simulink model "tb_kinematics"  (R2024b)
settings: Solver=VariableStepAuto  StartTime=0.0  StopTime=8  RelTol=1e-3
undefined symbols (not defined in the file): eta, ki_tuner, kp_tuner, openloop, Ts_s
libraries: slpidlib x2, simulink x1
settings Model: PacingRate=1.100000  Creator=icpmoles  LastModifiedBy=icpmoles

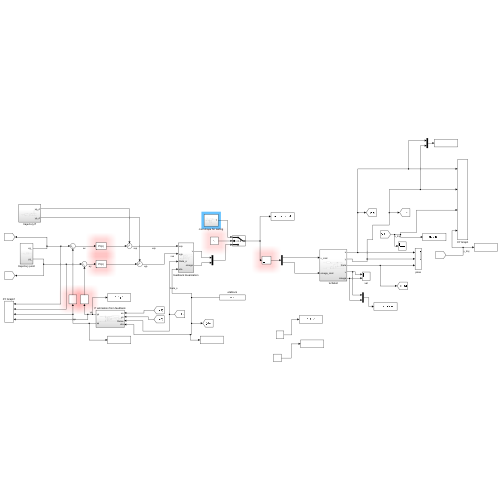
[thumbnail: Simulink's stored preview of the top-level diagram]
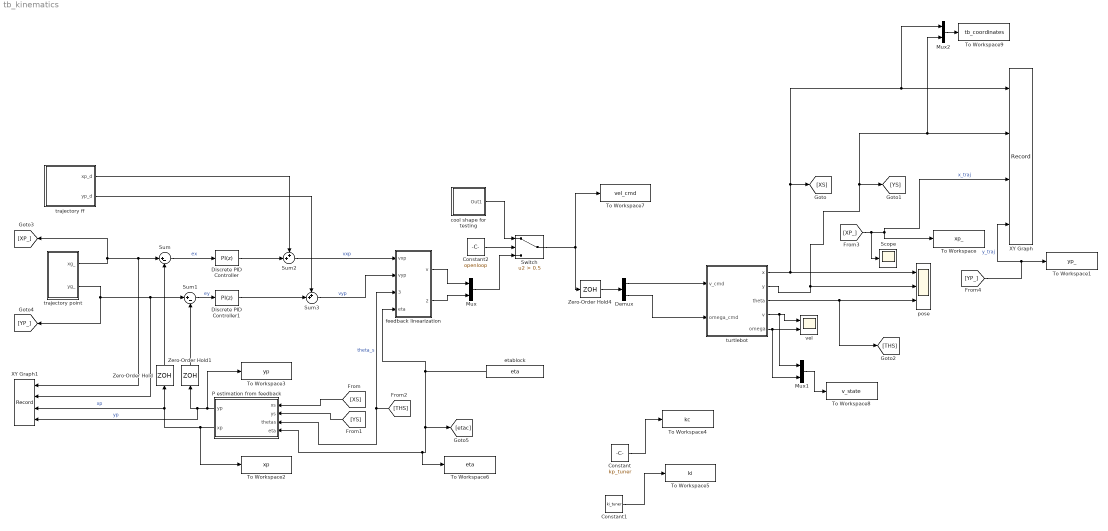
== system tb_kinematics ==
  Constant : Constant  Value=kp_tuner
  Constant1 : Constant  Value=ki_tuner
  Constant2 : Constant  Value=openloop
  Demux : Demux  Outputs=2
  Discrete PID Controller : slpidlib/PID Controller  Controller=PI  Form=Ideal  TimeDomain=Discrete-time  UseExternalTs=off  SampleTime=Ts_s  IntegratorMethod=Forward Euler  FilterMethod=Forward Euler  ControllerParametersSource=internal  P=kp_tuner  I=ki_tuner  UseKiTs=off  D=0  UseExternalDerivativeSource=off  N=100  UseFilter=on  TunerSelectOption=Transfer Function Based (PID Tuner App)  InitialConditionSource=internal  InitialConditionForIntegrator=0  InitialConditionForFilter=0  DifferentiatorICPrevScaledInput=0  ExternalReset=none  TrackingMode=off  Kt=1  LimitOutput=off  SatLimitsSource=internal  UpperSaturationLimit=inf  LowerSaturationLimit=-inf  LinearizeAsGain=off  AntiWindupMode=none  Kb=1  LimitIntegrator=off  UpperIntegratorSaturationLimit=inf  LowerIntegratorSaturationLimit=-inf  POutMin=[]  POutMax=[]  IOutMin=[]  IOutMax=[]  DOutMin=[]  DOutMax=[]  NOutMin=[]  NOutMax=[]  SumOutMin=[]  SumOutMax=[]  SaturationOutMin=[]  SaturationOutMax=[]  PParamMin=[]  PParamMax=[]  IParamMin=[]  IParamMax=[]  DParamMin=[]  DParamMax=[]  NParamMin=[]  NParamMax=[]  KbParamMin=[]  KbParamMax=[]  KtParamMin=[]  KtParamMax=[]  KbOutMin=[]  KbOutMax=[]  KtOutMin=[]  KtOutMax=[]  IntegratorOutMin=[]  IntegratorOutMax=[]  FilterOutMin=[]  FilterOutMax=[]  SumI1OutMin=[]  SumI1OutMax=[]  SumI2OutMin=[]  SumI2OutMax=[]  SumI3OutMin=[]  SumI3OutMax=[]  SumI4OutMin=[]  SumI4OutMax=[]  SumDOutMin=[]  SumDOutMax=[]  DifferentiatorOutMin=[]  DifferentiatorOutMax=[]  FilterDiffOutCoefMin=[]  FilterDiffOutCoefMax=[]  ReciprocalOutMin=[]  ReciprocalOutMax=[]  SumDenOutMin=[]  SumDenOutMax=[]  SumNumOutMin=[]  SumNumOutMax=[]  DivideOutMin=[]  DivideOutMax=[]  UdiffTsProdOutMin=[]  UdiffTsProdOutMax=[]  NTsProdOutMin=[]  NTsProdOutMax=[]  UintegralTsProdOutMin=[]  UintegralTsProdOutMax=[]  UngainTsProdOutMin=[]  UngainTsProdOutMax=[]  ClampingZeroOutDataTypeStr=Inherit: Inherit via back propagation  ClampingZeroOutMin=[]  ClampingZeroOutMax=[]  FilterDenConstantOutDataTypeStr=Inherit: Inherit via back propagation  FilterDenConstantOutMin=[]  FilterDenConstantOutMax=[]  PCopyOutDataTypeStr=Inherit: Inherit via back propagation  PCopyOutMin=[]  PCopyOutMax=[]  NCopyOutDataTypeStr=Inherit: Inherit via back propagation  NCopyOutMin=[]  NCopyOutMax=[]  IntegratorContinuousStateAttributes=''  IntegratorStateMustResolveToSignalObject=off  IntegratorRTWStateStorageClass=Auto  FilterContinuousStateAttributes=''  FilterStateMustResolveToSignalObject=off  FilterRTWStateStorageClass=Auto  ParallelPVariant=Passthrough  IdealPVariant=InternalParameters  IVariant=InternalParameters  DVariant=Disabled  IntegratorVariant=Discrete  SatVariant=Disabled  AWVariant=Passthrough  PCopyVariant=Disabled  TRVariant=Disabled  FdbkBlocksVariant=Forward  IdealPFdbkVariant=Disabled  SatFdbkVariant=Disabled  DerivativeFilterVariant=Disabled  NVariant=Disabled  NCopyVariant=Disabled_SignalSpec  FilterICVariant=Disabled  IntegratorICVariant=InternalICs  ExternalResetVariant=Disabled  TRSumVariant=Passthrough  SumFdbkVariant=Disabled  SumVariant=Sum_PI  TsampFilterVariant=InternalTs  TsampNgainVariant=Passthrough  TsampIntegralVariant=Disabled_SignalSpec  ExternalSaturationOutDataTypeStr=Inherit: Same as second input  DerivativeSourceVariant=Disabled  PreIntVariant=InternalPreInt
      settings: LibrarySourceBlock=hdlsllib/Discrete/Discrete PID Controller
  Discrete PID Controller1 : slpidlib/PID Controller  Controller=PI  Form=Ideal  TimeDomain=Discrete-time  UseExternalTs=off  SampleTime=Ts_s  IntegratorMethod=Forward Euler  FilterMethod=Forward Euler  ControllerParametersSource=internal  P=kp_tuner  I=ki_tuner  UseKiTs=off  D=0  UseExternalDerivativeSource=off  N=100  UseFilter=on  TunerSelectOption=Transfer Function Based (PID Tuner App)  InitialConditionSource=internal  InitialConditionForIntegrator=0  InitialConditionForFilter=0  DifferentiatorICPrevScaledInput=0  ExternalReset=none  TrackingMode=off  Kt=1  LimitOutput=off  SatLimitsSource=internal  UpperSaturationLimit=inf  LowerSaturationLimit=-inf  LinearizeAsGain=off  AntiWindupMode=none  Kb=1  LimitIntegrator=off  UpperIntegratorSaturationLimit=inf  LowerIntegratorSaturationLimit=-inf  POutMin=[]  POutMax=[]  IOutMin=[]  IOutMax=[]  DOutMin=[]  DOutMax=[]  NOutMin=[]  NOutMax=[]  SumOutMin=[]  SumOutMax=[]  SaturationOutMin=[]  SaturationOutMax=[]  PParamMin=[]  PParamMax=[]  IParamMin=[]  IParamMax=[]  DParamMin=[]  DParamMax=[]  NParamMin=[]  NParamMax=[]  KbParamMin=[]  KbParamMax=[]  KtParamMin=[]  KtParamMax=[]  KbOutMin=[]  KbOutMax=[]  KtOutMin=[]  KtOutMax=[]  IntegratorOutMin=[]  IntegratorOutMax=[]  FilterOutMin=[]  FilterOutMax=[]  SumI1OutMin=[]  SumI1OutMax=[]  SumI2OutMin=[]  SumI2OutMax=[]  SumI3OutMin=[]  SumI3OutMax=[]  SumI4OutMin=[]  SumI4OutMax=[]  SumDOutMin=[]  SumDOutMax=[]  DifferentiatorOutMin=[]  DifferentiatorOutMax=[]  FilterDiffOutCoefMin=[]  FilterDiffOutCoefMax=[]  ReciprocalOutMin=[]  ReciprocalOutMax=[]  SumDenOutMin=[]  SumDenOutMax=[]  SumNumOutMin=[]  SumNumOutMax=[]  DivideOutMin=[]  DivideOutMax=[]  UdiffTsProdOutMin=[]  UdiffTsProdOutMax=[]  NTsProdOutMin=[]  NTsProdOutMax=[]  UintegralTsProdOutMin=[]  UintegralTsProdOutMax=[]  UngainTsProdOutMin=[]  UngainTsProdOutMax=[]  ClampingZeroOutDataTypeStr=Inherit: Inherit via back propagation  ClampingZeroOutMin=[]  ClampingZeroOutMax=[]  FilterDenConstantOutDataTypeStr=Inherit: Inherit via back propagation  FilterDenConstantOutMin=[]  FilterDenConstantOutMax=[]  PCopyOutDataTypeStr=Inherit: Inherit via back propagation  PCopyOutMin=[]  PCopyOutMax=[]  NCopyOutDataTypeStr=Inherit: Inherit via back propagation  NCopyOutMin=[]  NCopyOutMax=[]  IntegratorContinuousStateAttributes=''  IntegratorStateMustResolveToSignalObject=off  IntegratorRTWStateStorageClass=Auto  FilterContinuousStateAttributes=''  FilterStateMustResolveToSignalObject=off  FilterRTWStateStorageClass=Auto  ParallelPVariant=Passthrough  IdealPVariant=InternalParameters  IVariant=InternalParameters  DVariant=Disabled  IntegratorVariant=Discrete  SatVariant=Disabled  AWVariant=Passthrough  PCopyVariant=Disabled  TRVariant=Disabled  FdbkBlocksVariant=Forward  IdealPFdbkVariant=Disabled  SatFdbkVariant=Disabled  DerivativeFilterVariant=Disabled  NVariant=Disabled  NCopyVariant=Disabled_SignalSpec  FilterICVariant=Disabled  IntegratorICVariant=InternalICs  ExternalResetVariant=Disabled  TRSumVariant=Passthrough  SumFdbkVariant=Disabled  SumVariant=Sum_PI  TsampFilterVariant=InternalTs  TsampNgainVariant=Passthrough  TsampIntegralVariant=Disabled_SignalSpec  ExternalSaturationOutDataTypeStr=Inherit: Same as second input  DerivativeSourceVariant=Disabled  PreIntVariant=InternalPreInt
      settings: LibrarySourceBlock=hdlsllib/Discrete/Discrete PID Controller
  Mux : Mux  Inputs=2
  Mux1 : Mux  Inputs=2
  Mux2 : Mux  Inputs=2
  P estimation from feedback : Subsystem
  Scope : Scope
  Sum : Sum  Inputs=|+-
  Sum1 : Sum  Inputs=|+-
  Sum2 : Sum  Inputs=++|
  Sum3 : Sum  Inputs=++|
  Switch : Switch  Criteria=u2 > Threshold  Threshold=0.5  SaturateOnIntegerOverflow=off  InputSameDT=off
  To Workspace : ToWorkspace  VariableName=xp_  SaveFormat=Timeseries  SampleTime=-1
  To Workspace1 : ToWorkspace  VariableName=yp_  SaveFormat=Timeseries  SampleTime=-1
  To Workspace2 : ToWorkspace  VariableName=xp  SaveFormat=Timeseries  SampleTime=-1
  To Workspace3 : ToWorkspace  VariableName=yp  SaveFormat=Timeseries  SampleTime=-1
  To Workspace4 : ToWorkspace  VariableName=kc  SaveFormat=Timeseries  SampleTime=-1
  To Workspace5 : ToWorkspace  VariableName=ki  SaveFormat=Timeseries  SampleTime=-1
  To Workspace6 : ToWorkspace  VariableName=eta  SaveFormat=Timeseries  SampleTime=-1
  To Workspace7 : ToWorkspace  VariableName=vel_cmd  SaveFormat=Timeseries  SampleTime=-1
  To Workspace8 : ToWorkspace  VariableName=v_state  SaveFormat=Timeseries  SampleTime=-1
  To Workspace9 : ToWorkspace  VariableName=tb_coordinates  SaveFormat=Timeseries  SampleTime=-1
  XY Graph : Record  FileSettingsInternal="{\"entries\":[{\"content\":{\"excelSettings\":{\"content\":{},\"type\":\"Streamout.ExcelSettings\"}},\"type\":\"Streamout.FileSettingStorage\",\"uuid\":\"\"}],\"packageUris\":[\"http:\\/\\/schema.mathworks.com\\/mf0\\/streamout_blocks\\/R2020a\"],\"version\":\"1.0\"}"  Layout=[1 1]  SignalsInternal="{\"entries\":[{\"content\":{\"signals\":[{\"content\":{\"blockPath\":[],\"dimensions\":[1],\"domain\":\"\",\"lineColor\":\"#a2142f\",\"plots\":[ 1 ],\"port\":1,\"sid\":[\"\"],\"signalID\":1,\"signalName\":\"turtlebot:1\"},\"type\":\"RecordBlkView.Signal\",\"uuid\":\"\"},{\"content\":{\"blockPath\":[],\"dimensions\":[1],\"domain\":\"\",\"lineColor\":\"#139fff\",\"plots\":[ 1 ],\"port\":2,\"sid\":[\"\"],\"signalID\":2,\"signalName\":\"turtlebot:2\"},\"type\":\"RecordBlkView.Signal\",\"uuid\":\"\"},{\"content\":{\"blockPath\":[],\"dimensions\":[1],\"domain\":\"\",\"lineColor\":\"#64d413\",\"lineWidth\":2,\"plots\":[ 1 ],\"port\":3,\"sid\":[\"\"],\"signalID\":3,\"signalName\":\"x_traj\"},\"type\":\"RecordBlkView.Signal\",\"uuid\":\"\"},{\"content\":{\"blockPath\":[],\"dimensions\":[1],\"domain\":\"\",\"lineColor\":\"#ff13a6\",\"lineWidth\":2,\"plots\":[ 1 ],\"port\":4,\"sid\":[\"\"],\"signalID\":4,\"signalName\":\"y_traj\"},\"type\":\"RecordBlkView.Signal\",\"uuid\":\"\"}]},\"type\":\"RecordBlkView.InputSignals\",\"uuid\":\"\"}],\"packageUris\":[\"http:\\/\\/schema.mathworks.com\\/mf0\\/streamout_blocks\\/R2020a\"],\"version\":\"1.0\"}"  VisualizationBindings="{\"xyplotplugin\":{\"info\":[{\"series\":[{\"bindingParametersList\":[{\"parameter\":\"X-Axis\",\"signalID\":1,\"signalName\":\"turtlebot:1\"},{\"parameter\":\"Y-Axis\",\"signalID\":2,\"signalName\":\"turtlebot:2\"}],\"seriesID\":0},{\"bindingParametersList\":[{\"parameter\":\"X-Axis\",\"signalID\":3,\"signalName\":\"x_traj\"},{\"parameter\":\"Y-Axis\",\"signalID\":4,\"signalName\":\"y_traj\"}],\"seriesID\":1}],\"subplotID\":1},{\"series\":[],\"subplotID\":9}]}}"  CompatibilityTag=XY
  XY Graph1 : Record  FileSettingsInternal="{\"entries\":[{\"content\":{\"excelSettings\":{\"content\":{},\"type\":\"Streamout.ExcelSettings\"}},\"type\":\"Streamout.FileSettingStorage\",\"uuid\":\"\"}],\"packageUris\":[\"http:\\/\\/schema.mathworks.com\\/mf0\\/streamout_blocks\\/R2020a\"],\"version\":\"1.0\"}"  Layout=[1 1]  SignalsInternal="{\"entries\":[{\"content\":{\"signals\":[{\"content\":{\"blockPath\":[],\"dimensions\":[1],\"domain\":\"\",\"lineColor\":\"#a2142f\",\"plots\":[ 1 ],\"port\":1,\"sid\":[\"\"],\"signalID\":1,\"signalName\":\"trajectory point:1\"},\"type\":\"RecordBlkView.Signal\",\"uuid\":\"\"},{\"content\":{\"blockPath\":[],\"dimensions\":[1],\"domain\":\"\",\"lineColor\":\"#139fff\",\"plots\":[ 1 ],\"port\":2,\"sid\":[\"\"],\"signalID\":2,\"signalName\":\"trajectory point:2\"},\"type\":\"RecordBlkView.Signal\",\"uuid\":\"\"},{\"content\":{\"blockPath\":[],\"dimensions\":[1],\"domain\":\"\",\"lineColor\":\"#edb120\",\"lineWidth\":2,\"plots\":[ 1 ],\"port\":3,\"sid\":[\"\"],\"signalID\":3,\"signalName\":\"xp\"},\"type\":\"RecordBlkView.Signal\",\"uuid\":\"\"},{\"content\":{\"blockPath\":[],\"dimensions\":[1],\"domain\":\"\",\"lineColor\":\"#7e2f8e\",\"lineWidth\":2,\"plots\":[ 1 ],\"port\":4,\"sid\":[\"\"],\"signalID\":4,\"signalName\":\"yp\"},\"type\":\"RecordBlkView.Signal\",\"uuid\":\"\"}]},\"type\":\"RecordBlkView.InputSignals\",\"uuid\":\"\"}],\"packageUris\":[\"http:\\/\\/schema.mathworks.com\\/mf0\\/streamout_blocks\\/R2020a\"],\"version\":\"1.0\"}"  VisualizationBindings="{\"xyplotplugin\":{\"info\":[{\"series\":[{\"bindingParametersList\":[{\"parameter\":\"X-Axis\",\"signalID\":1,\"signalName\":\"trajectory point:1\"},{\"parameter\":\"Y-Axis\",\"signalID\":2,\"signalName\":\"trajectory point:2\"}],\"seriesID\":0},{\"bindingParametersList\":[{\"parameter\":\"X-Axis\",\"signalID\":3,\"signalName\":\"xp\"},{\"parameter\":\"Y-Axis\",\"signalID\":4,\"signalName\":\"yp\"}],\"seriesID\":1}],\"subplotID\":1}]}}"  CompatibilityTag=XY
  Zero-Order Hold : ZeroOrderHold  SampleTime=Ts_s
  Zero-Order Hold1 : ZeroOrderHold  SampleTime=Ts_s
  Zero-Order Hold4 : ZeroOrderHold  SampleTime=Ts_s
  cool shape for testing : Subsystem
  etablock : Constant  Value=eta
  feedback linearization : Subsystem
  pose : Scope  NumInputPorts=3
  trajectory ff : Subsystem
  trajectory point : Subsystem
  turtlebot : Subsystem
  vel : Scope  NumInputPorts=2
  wires:
  turtlebot/1(x) -> [XS], Mux2/1, XY Graph/1, pose/1
  turtlebot/3(theta) -> [THS], pose/3
  turtlebot/4(v) -> Mux1/1, vel/1
  turtlebot/5(omega) -> Mux1/2, vel/2
  Demux/1 -> turtlebot/1(v_cmd)
  Demux/2 -> turtlebot/2(omega_cmd)
  P estimation from feedback/2(xp) -> To Workspace2/1, Zero-Order Hold/1, XY Graph1/3  "xp"
  P estimation from feedback/1(yp) -> To Workspace3/1, XY Graph1/4, Zero-Order Hold1/1  "yp"
  trajectory point/2(yg_) -> [YP_], XY Graph1/2, Sum1/1
  Sum/1 -> Discrete PID Controller/1  "ex"
  Sum1/1 -> Discrete PID Controller1/1  "ey"
  Discrete PID Controller1/1 -> Sum3/2
  Discrete PID Controller/1 -> Sum2/2
  [XS] -> P estimation from feedback/1(xs)
  [YS] -> P estimation from feedback/2(ys)
  [THS] -> P estimation from feedback/3(thetas), feedback linearization/3(theta_s)  "theta_s"
  Sum2/1 -> feedback linearization/1(vxp)  "vxp"
  Sum3/1 -> feedback linearization/2(vyp)  "vyp"
  etablock/1 -> [etac], To Workspace6/1, P estimation from feedback/4(eta), feedback linearization/4(eta)
  trajectory ff/2(yp_d) -> Sum3/1
  trajectory ff/1(xp_d) -> Sum2/1
  Zero-Order Hold/1 -> Sum/2
  Zero-Order Hold1/1 -> Sum1/2
  trajectory point/1(xg_) -> [XP_], XY Graph1/1, Sum/1
  [XP_] -> Scope/1, To Workspace/1, XY Graph/3  "x_traj"
  [YP_] -> XY Graph/4, To Workspace1/1  "y_traj"
  Constant/1 -> To Workspace4/1
  Constant1/1 -> To Workspace5/1
  feedback linearization/1(v) -> Mux/1
  feedback linearization/2(omega) -> Mux/2
  Constant2/1 -> Switch/2
  Zero-Order Hold4/1 -> Demux/1
  Mux/1 -> Switch/3
  cool shape for testing/1(Out1) -> Switch/1
  Mux1/1 -> To Workspace8/1
  Mux2/1 -> To Workspace9/1
  turtlebot/2(y) -> [YS], Mux2/2, XY Graph/2, pose/2
  Switch/1 -> Zero-Order Hold4/1, To Workspace7/1

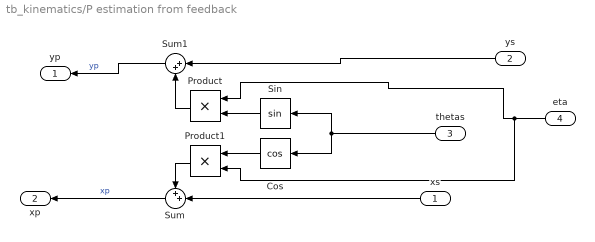
== system tb_kinematics/P estimation from feedback ==
  xs : Inport
  ys : Inport  Port=2
  thetas : Inport  Port=3
  eta : Inport  Port=4
  Cos : Trigonometry  Operator=cos
  Product : Product
  Product1 : Product
  Sin : Trigonometry
  Sum : Sum  Inputs=++|
  Sum1 : Sum  Inputs=|++
  yp : Outport
  xp : Outport  Port=2
  wires:
  xs/1 -> Sum/2
  thetas/1 -> Sin/1, Cos/1
  Sum/1 -> xp/1  "xp"
  Product1/1 -> Sum/1
  ys/1 -> Sum1/1
  Sin/1 -> Product/2
  Sum1/1 -> yp/1  "yp"
  Product/1 -> Sum1/2
  Cos/1 -> Product1/1
  eta/1 -> Product1/2, Product/1

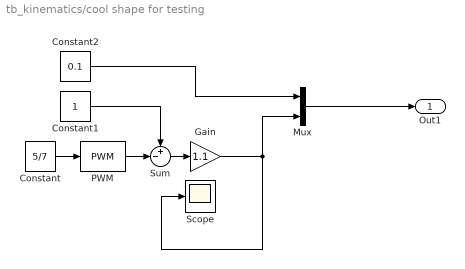
== system tb_kinematics/cool shape for testing ==
  Constant : Constant  Value=5/7
  Constant1 : Constant
  Constant2 : Constant  Value=0.1
  Gain : Gain  Gain=1.1
  Mux : Mux  Inputs=2
  PWM : simulink/Discontinuities/PWM  DisableCoverage=on  Period=7  InitialDelay=0  DisallowZeroDutyCycle=off  RunAtFixedTimeIntervals=off  SampleTime=0.1
  Scope : Scope
  Sum : Sum  Inputs=+-|
  Out1 : Outport
  wires:
  PWM/1 -> Sum/2
  Gain/1 -> Mux/2, Scope/1
  Constant1/1 -> Sum/1
  Constant/1 -> PWM/1
  Constant2/1 -> Mux/1
  Sum/1 -> Gain/1
  Mux/1 -> Out1/1

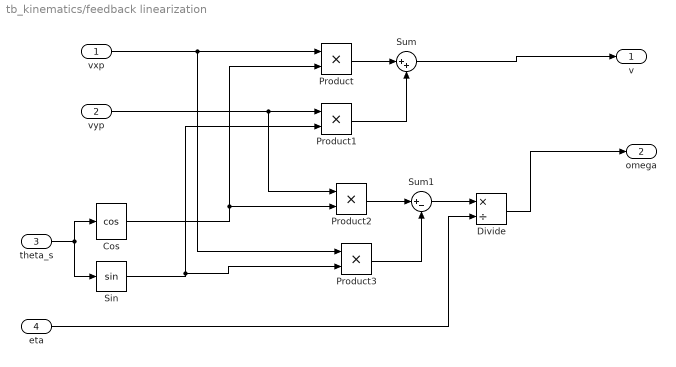
== system tb_kinematics/feedback linearization ==
  vxp : Inport
  vyp : Inport  Port=2
  theta_s : Inport  Port=3
  eta : Inport  Port=4
  Cos : Trigonometry  Operator=cos
  Divide : Product  Inputs=*/
  Product{,1..3} (4 alike) : Product
  Sin : Trigonometry
  Sum : Sum  Inputs=|++
  Sum1 : Sum  Inputs=|+-
  v : Outport
  omega : Outport  Port=2
  wires:
  theta_s/1 -> Sin/1, Cos/1
  vyp/1 -> Product2/1, Product1/1
  vxp/1 -> Product3/1, Product/1
  Cos/1 -> Product/2, Product2/2
  Product/1 -> Sum/1
  Sin/1 -> Product3/2, Product1/2
  Product1/1 -> Sum/2
  Product2/1 -> Sum1/1
  Product3/1 -> Sum1/2
  Sum1/1 -> Divide/1
  Divide/1 -> omega/1
  Sum/1 -> v/1
  eta/1 -> Divide/2

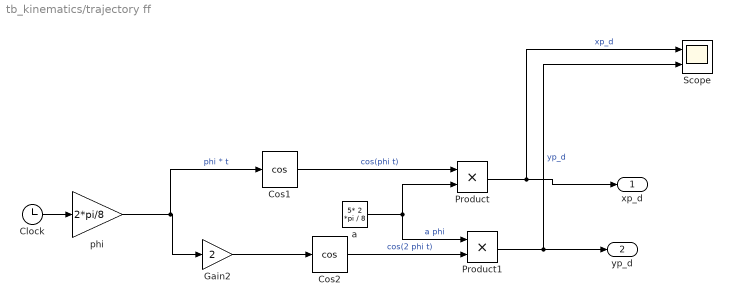
== system tb_kinematics/trajectory ff ==
  Clock : Clock
  Cos1 : Trigonometry  Operator=cos
  Cos2 : Trigonometry  Operator=cos
  Gain2 : Gain  Gain=2
  Product : Product
  Product1 : Product
  Scope : Scope  NumInputPorts=2
  a : Constant  Value=5* 2 *pi / 8
  phi : Gain  Gain=2*pi/8
  xp_d : Outport
  yp_d : Outport  Port=2
  wires:
  Product/1 -> Scope/1, xp_d/1  "xp_d"
  Cos1/1 -> Product/1  "cos(phi t)"
  Product1/1 -> Scope/2, yp_d/1  "yp_d"
  Clock/1 -> phi/1
  Cos2/1 -> Product1/2  "cos(2 phi t)"
  phi/1 -> Cos1/1, Gain2/1  "phi * t"
  a/1 -> Product1/1, Product/2  "a phi"
  Gain2/1 -> Cos2/1

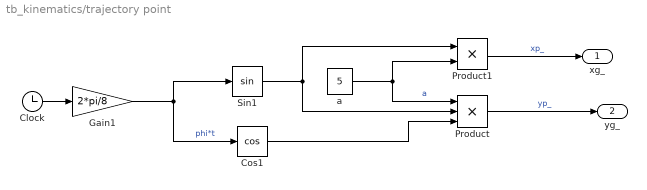
== system tb_kinematics/trajectory point ==
  Clock : Clock
  Cos1 : Trigonometry  Operator=cos
  Gain1 : Gain  Gain=2*pi/8
  Product : Product  Inputs=3
  Product1 : Product
  Sin1 : Trigonometry
  a : Constant  Value=5
  xg_ : Outport
  yg_ : Outport  Port=2
  wires:
  Gain1/1 -> Cos1/1, Sin1/1  "phi*t"
  Product1/1 -> xg_/1  "xp_"
  a/1 -> Product/1, Product1/2  "a"
  Sin1/1 -> Product/2, Product1/1
  Cos1/1 -> Product/3
  Clock/1 -> Gain1/1
  Product/1 -> yg_/1  "yp_"

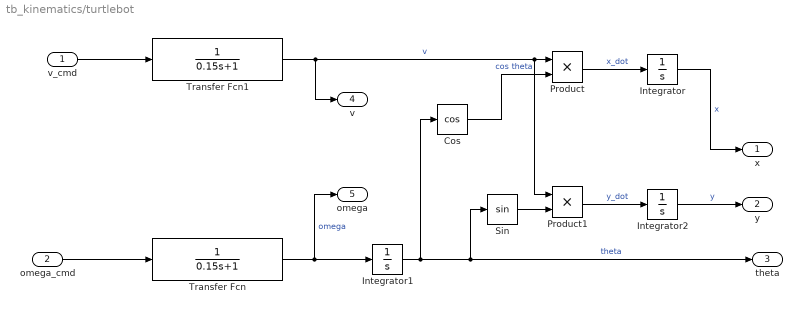
== system tb_kinematics/turtlebot ==
  v_cmd : Inport
  omega_cmd : Inport  Port=2
  Cos : Trigonometry  Operator=cos
  Integrator : Integrator
  Integrator1 : Integrator
  Integrator2 : Integrator
  Product : Product
  Product1 : Product
  Sin : Trigonometry
  Transfer Fcn : TransferFcn  Denominator=[0.15 1]
  Transfer Fcn1 : TransferFcn  Denominator=[0.15 1]
  x : Outport
  y : Outport  Port=2
  theta : Outport  Port=3
  v : Outport  Port=4
  omega : Outport  Port=5
  wires:
  Transfer Fcn/1 -> omega/1, Integrator1/1  "omega"
  Transfer Fcn1/1 -> Product1/1, Product/1, v/1  "v"
  v_cmd/1 -> Transfer Fcn1/1
  Product/1 -> Integrator/1  "x_dot"
  omega_cmd/1 -> Transfer Fcn/1
  Product1/1 -> Integrator2/1  "y_dot"
  Integrator1/1 -> theta/1, Sin/1, Cos/1  "theta"
  Cos/1 -> Product/2  "cos theta"
  Sin/1 -> Product1/2
  Integrator/1 -> x/1  "x"
  Integrator2/1 -> y/1  "y"
